simulink model "lab2"  (R2021a)
settings: Solver=VariableStepAuto  StartTime=0.0  StopTime=50  MaxStep=0.001  RelTol=1e-3
settings Model: Creator=asr77  LastModifiedBy=asr77

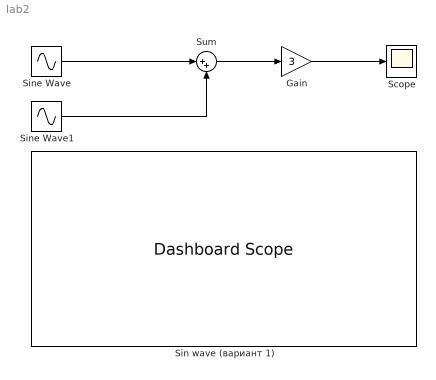
== system lab2 ==
  Gain : Gain  Gain=3
  Scope : Scope
  Sin wave (вариант 1) : DashboardScope  LegendPosition=Hide
  Sine Wave : Sin  Amplitude=1:1:4  SampleTime=0
  Sine Wave1 : Sin  Amplitude=0.05  Frequency=10  SampleTime=0
  Sum : Sum  Inputs=|++
  wires:
  Gain/1 -> Scope/1
  Sine Wave/1 -> Sum/1
  Sine Wave1/1 -> Sum/2
  Sum/1 -> Gain/1
